simulink model "magnetic_field"  (R2023b)
settings: Solver=VariableStepAuto  StartTime=0.0  StopTime=10.0  RelTol=1e-3
undefined symbols (not defined in the file or in its folder): A1, A2, n_earth, timeoflaunch
libraries: simulink_extras x1, matrix_library x1
settings Model: Creator=edoardonicolucci  LastModifiedBy=edoardonicolucci

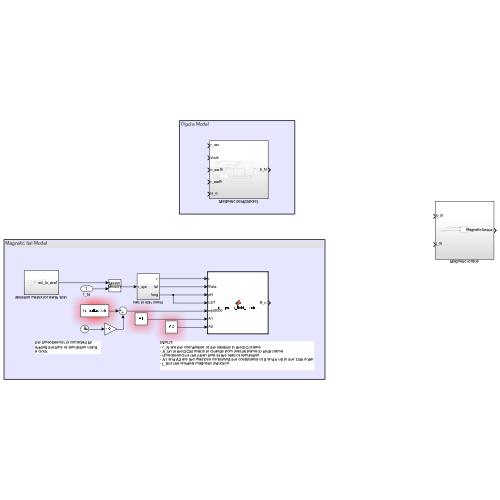
[thumbnail: Simulink's stored preview of the top-level diagram]
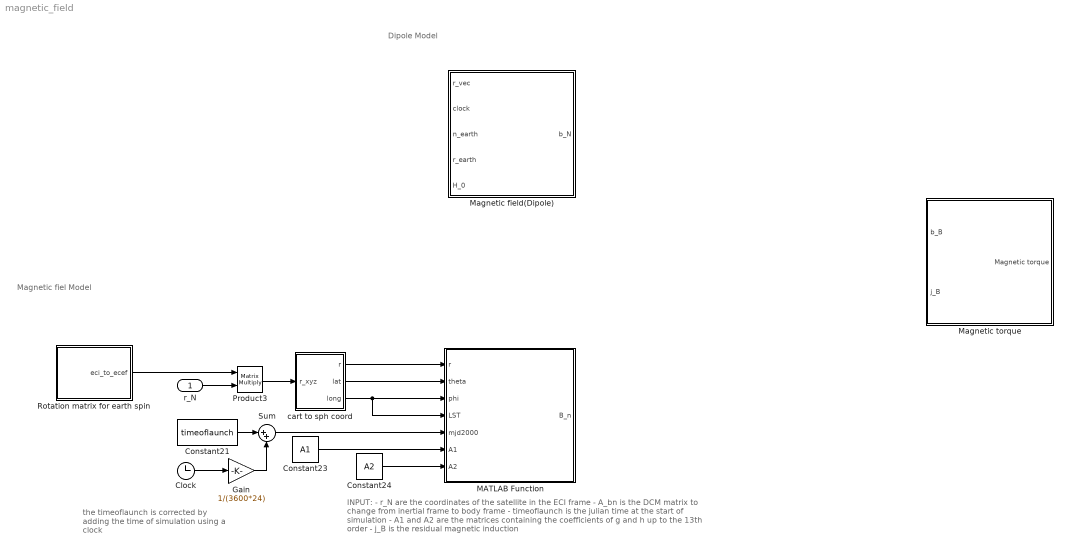
== system magnetic_field ==
  note: Dipole Model
  note: Magnetic fiel Model
  note: INPUT:
      | - r_N are the coordinates of the satellite in the ECI frame
      | - A_bn is the DCM matrix to change from inertial frame to body frame
      | - timeoflaunch is the julian time at the start of simulation
      | - A1 and A2 are the matrices containing the coefficients of g and h up to the 13th order
      | - j_B is the residual magnetic induction
  note: the timeoflaunch is corrected by adding the time of simulation using a clock
  r_N : Inport
  Clock : Clock
  Constant21 : Constant  Value=timeoflaunch
  Constant23 : Constant  Value=A1
  Constant24 : Constant  Value=A2
  Gain : Gain  Gain=1/(3600*24)
  MATLAB Function : MATLAB Function  TreatAsAtomicUnit=on
  Magnetic field(Dipole) : Subsystem
  Magnetic torque : Subsystem
  Product3 : Product  Multiplication=Matrix(*)
  Rotation matrix for earth spin : Subsystem
  Sum : Sum  Inputs=|++
  cart to sph coord : Subsystem
  wires:
  cart to sph coord/3(long) -> MATLAB Function/4(LST), MATLAB Function/3(phi)
  Constant23/1 -> MATLAB Function/6(A1)
  Product3/1 -> cart to sph coord/1(r_xyz)
  cart to sph coord/2(lat) -> MATLAB Function/2(theta)
  Constant24/1 -> MATLAB Function/7(A2)
  r_N/1 -> Product3/2
  Clock/1 -> Gain/1
  Rotation matrix for earth spin/1(eci_to_ecef) -> Product3/1
  Constant21/1 -> Sum/1
  Sum/1 -> MATLAB Function/5(mjd2000)
  cart to sph coord/1(r) -> MATLAB Function/1(r)
  Gain/1 -> Sum/2

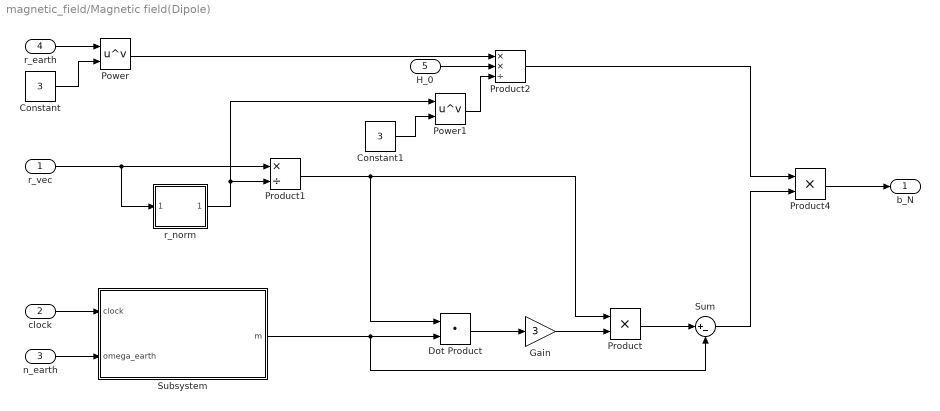
== system magnetic_field/Magnetic field(Dipole) ==
  r_vec : Inport
  clock : Inport  Port=2
  n_earth : Inport  Port=3
  r_earth : Inport  Port=4
  H_0 : Inport  Port=5
  Constant : Constant  Value=3
  Constant1 : Constant  Value=3
  Dot Product : DotProduct  OutDataTypeStr=Inherit: Inherit via internal rule
  Gain : Gain  Gain=3
  Power : Math  Operator=pow
  Power1 : Math  Operator=pow
  Product : Product
  Product1 : Product  Inputs=*/
  Product2 : Product  Inputs=**/
  Product4 : Product
  Subsystem : Subsystem
  Sum : Sum  Inputs=|+-
  r_norm : Subsystem
  b_N : Outport
  wires:
  Gain/1 -> Product/2
  Sum/1 -> Product4/2
  n_earth/1 -> Subsystem/2(omega_earth)
  clock/1 -> Subsystem/1(clock)
  Subsystem/1(m) -> Dot Product/2, Sum/2
  Product/1 -> Sum/1
  Dot Product/1 -> Gain/1
  r_vec/1 -> Product1/1, r_norm/1(Input)
  r_norm/1(Output) -> Power1/1, Product1/2
  Product1/1 -> Product/1, Dot Product/1
  r_earth/1 -> Power/1
  Constant/1 -> Power/2
  Power/1 -> Product2/1
  H_0/1 -> Product2/2
  Product2/1 -> Product4/1
  Product4/1 -> b_N/1
  Constant1/1 -> Power1/2
  Power1/1 -> Product2/3

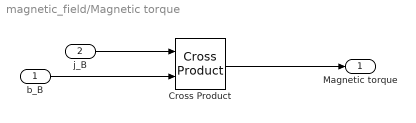
== system magnetic_field/Magnetic torque ==
  b_B : Inport
  j_B : Inport  Port=2
  Cross Product : matrix_library/Cross Product
  Magnetic torque : Outport
  wires:
  j_B/1 -> Cross Product/1
  b_B/1 -> Cross Product/2
  Cross Product/1 -> Magnetic torque/1

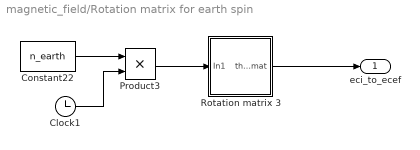
== system magnetic_field/Rotation matrix for earth spin ==
  Clock1 : Clock
  Constant22 : Constant  Value=n_earth
  Product3 : Product
  Rotation matrix 3 : Subsystem
  eci_to_ecef : Outport
  wires:
  Rotation matrix 3/1(theta_mat) -> eci_to_ecef/1
  Product3/1 -> Rotation matrix 3/1(In1)
  Constant22/1 -> Product3/1
  Clock1/1 -> Product3/2

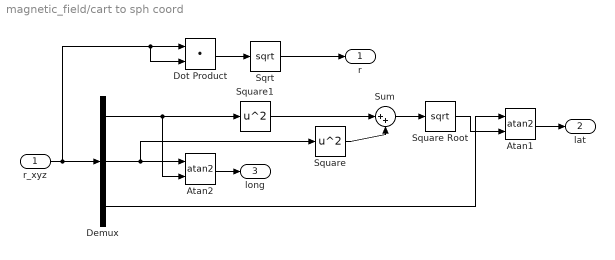
== system magnetic_field/cart to sph coord ==
  r_xyz : Inport
  Atan1 : Trigonometry  Operator=atan2
  Atan2 : Trigonometry  Operator=atan2
  Demux : Demux  Outputs=3
  Dot Product : DotProduct  OutDataTypeStr=Inherit: Inherit via internal rule
  Sqrt : Sqrt
  Square : Math  Operator=square
  Square Root : Sqrt
  Square1 : Math  Operator=square
  Sum : Sum  Inputs=|++
  r : Outport
  lat : Outport  Port=2
  long : Outport  Port=3
  wires:
  r_xyz/1 -> Dot Product/2, Dot Product/1, Demux/1
  Demux/2 -> Square/1, Atan2/1
  Demux/1 -> Atan2/2, Square1/1
  Atan2/1 -> long/1
  Demux/3 -> Atan1/1
  Square1/1 -> Sum/1
  Square/1 -> Sum/2
  Sum/1 -> Square Root/1
  Square Root/1 -> Atan1/2
  Atan1/1 -> lat/1
  Dot Product/1 -> Sqrt/1
  Sqrt/1 -> r/1

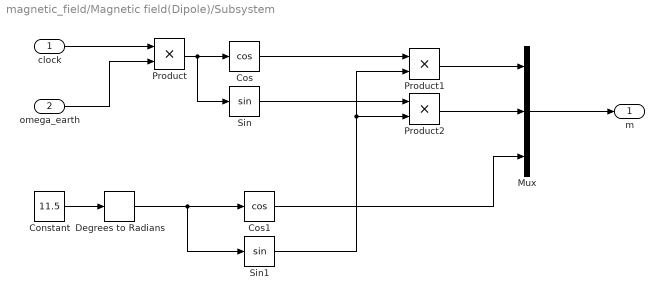
== system magnetic_field/Magnetic field(Dipole)/Subsystem ==
  clock : Inport
  omega_earth : Inport  Port=2
  Constant : Constant  Value=11.5
  Cos : Trigonometry  Operator=cos
  Cos1 : Trigonometry  Operator=cos
  Degrees to Radians : simulink_extras/Transformations/Degrees to Radians
  Mux : Mux  Inputs=3
  Product : Product
  Product1 : Product
  Product2 : Product
  Sin : Trigonometry
  Sin1 : Trigonometry
  m : Outport
  wires:
  clock/1 -> Product/1
  omega_earth/1 -> Product/2
  Product/1 -> Sin/1, Cos/1
  Constant/1 -> Degrees to Radians/1
  Degrees to Radians/1 -> Sin1/1, Cos1/1
  Sin1/1 -> Product2/2, Product1/2
  Cos/1 -> Product1/1
  Sin/1 -> Product2/1
  Cos1/1 -> Mux/3
  Product2/1 -> Mux/2
  Product1/1 -> Mux/1
  Mux/1 -> m/1

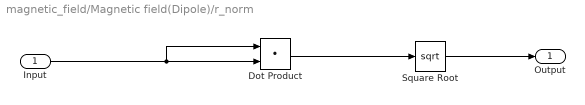
== system magnetic_field/Magnetic field(Dipole)/r_norm ==
  Input : Inport
  Dot Product : DotProduct  OutDataTypeStr=Inherit: Inherit via internal rule
  Square Root : Sqrt
  Output : Outport
  wires:
  Square Root/1 -> Output/1
  Dot Product/1 -> Square Root/1
  Input/1 -> Dot Product/1, Dot Product/2

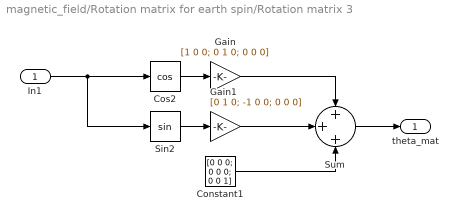
== system magnetic_field/Rotation matrix for earth spin/Rotation matrix 3 ==
  In1 : Inport
  Constant1 : Constant  Value=[0 0 0; 0 0 0; 0 0 1]
  Cos2 : Trigonometry  Operator=cos
  Gain : Gain  Gain=[1 0 0; 0 1 0; 0 0 0]
  Gain1 : Gain  Gain=[0 1 0; -1 0 0; 0 0 0]
  Sin2 : Trigonometry
  Sum : Sum  Inputs=+++
  theta_mat : Outport
  wires:
  Cos2/1 -> Gain/1
  Gain/1 -> Sum/1
  In1/1 -> Sin2/1, Cos2/1
  Sin2/1 -> Gain1/1
  Sum/1 -> theta_mat/1
  Gain1/1 -> Sum/2
  Constant1/1 -> Sum/3

== matlab function magnetic_field/MATLAB Function ==
  data: r input; B_n output; theta input; phi input; LST input; mjd2000 input; A1 input; A2 input
function B_n = magnetic_field_model(r,theta,phi, LST, mjd2000, A1, A2)

%   mjd2000[1]  Date in MJD 2000. MJD2000 is defined as the number of days
%               since 01-01-2000, 12:00 noon.
days = mjd2000 - 7305;      % 7305 is the Julian time from 2000 to 2020

% Inputs
% r         Geocentric radius
% theta     Latitude measured in degrees positive from equator  
% phi       Longitude measured in degrees positive east from Greenwich
% days      Decimal days since January 1, 2020
%
% Outputs - magnetic field strength in local tangential coordinates
% Br    B in radial direction
% Bt    B in theta direction
% Bp    B in phi direction
[Br,Bt,Bp] = magnet(r,theta,phi,days, A1, A2);

% Inputs
% Br    B in radial direction
% Bt    B in theta direction
% Bp    B in phi direction
% LST   Local sidereal time of location (in degrees)(right ascension)
% lat   Latitude measured positive north from equator (in degrees), it is
%       the same as the local declination
%
% Outputs
% Bx    B in x-direction  | Magnetic field strength (B)
% By    B in y-direction  | in geocentric inertial coordinates
% Bz    B in z-direction  |
[Bx,By,Bz] = msph2inert(Br,Bt,Bp,LST, theta);

B_n = [Bx,By,Bz]';
